simulink model "Lab6_3"  (R2021a)
settings: Solver=VariableStepAuto  StartTime=0.0  StopTime=.07  RelTol=1e-3  EnableMultiTasking=on
libraries: spsIGBTDiodeLib x8, spsDCVoltageSourceLib x2, spsTriangleGeneratorLib x2, spsSeriesRLCBranchLib x1, spsVoltageMeasurementLib x1, spspowerguiLib x1
settings Model: Creator=usee  LastModifiedBy=User
settings SolverCC: AlgebraicLoopSolver=TrustRegion
settings DataIOCC: ReturnWorkspaceOutputs=off
settings OptimizationCC: LifeSpan=inf
settings DebuggingCC: SFUnexpectedBacktrackingDiag=warning  SFNoUnconditionalDefaultTransitionDiag=warning  SFMachineParentedDataDiag=warning  ArithmeticOperatorsInVariantConditions=warning
settings SFSimCC: SimUseLocalCustomCode=off  CustomCodeUndefinedFunction=UseInterfaceOnly
settings RTWCC: RTWUseLocalCustomCode=off
settings CodeAppCC: StateflowObjectComments=on
settings GRTTargetCC: TargetLangStandard=C89/C90 (ANSI)
settings ConfigComp: CovMetricSettings=dw  CovSaveCumulativeToWorkspaceVar=on  CovSaveSingleToWorkspaceVar=on  CovExternalEMLEnable=off
settings SimscapeCC: SimscapeNormalizeSystem=off

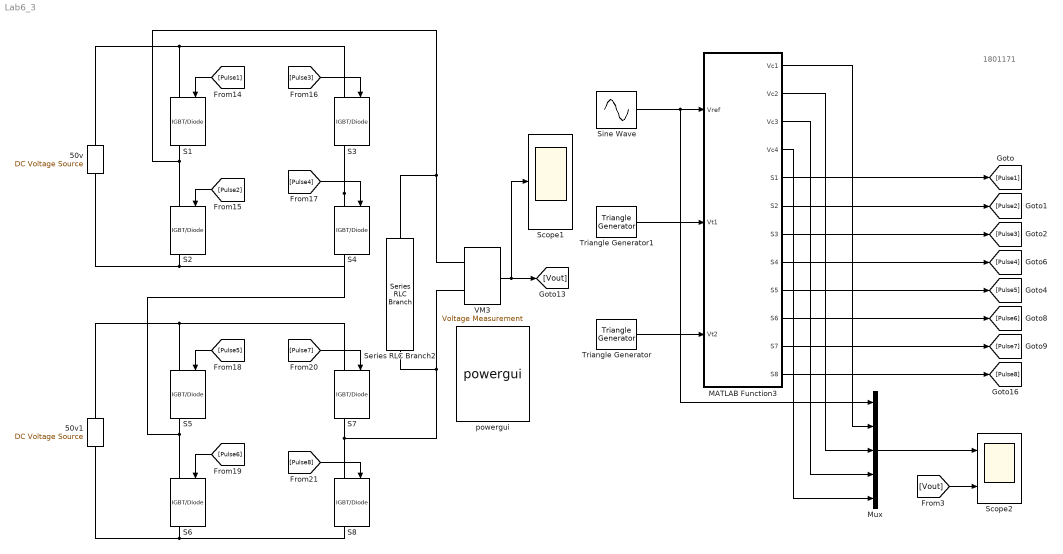
== system Lab6_3 ==
  note: 1801171
  50v : spsDCVoltageSourceLib/DC Voltage Source  Amplitude=50  Measurements=None
  50v1 : spsDCVoltageSourceLib/DC Voltage Source  Amplitude=50  Measurements=None
  MATLAB Function3 : MATLAB Function  TreatAsAtomicUnit=on
  Mux : Mux  Inputs=5
  S{1..8} (8 alike) : spsIGBTDiodeLib/IGBT//Diode  Ron=1e-3  Rs=1e5  Cs=inf  Measurements=on
  Scope1 : Scope
  Scope2 : Scope  NumInputPorts=2
  Series RLC Branch2 : spsSeriesRLCBranchLib/Series RLC Branch  LConnTagsString=__new0  RConnTagsString=__new0  BranchType=RL  Resistance=5  Inductance=10e-3  SetiL0=off  InitialCurrent=0  Capacitance=1e-6  Setx0=off  InitialVoltage=0  Measurements=None
  Sine Wave : Sin  Frequency=2*pi*50  SampleTime=0
  Triangle Generator : spsTriangleGeneratorLib/Triangle Generator  Freq=1000  Phase=0  Ts=0
  Triangle Generator1 : spsTriangleGeneratorLib/Triangle Generator  Freq=1000  Phase=180  Ts=0
  VM3 : spsVoltageMeasurementLib/Voltage Measurement  PhasorSimulation=off  OutputType=Complex  PSBequivalent=0
  powergui : spspowerguiLib/powergui  Priority=1  SimulationMode=Discrete  SampleTime=50e-6  frequency=60  Iterations=50  frequencyindice=0  Pbase=100e6  ErrMax=1e-4  UnitsV=kV  UnitsW=MW  buscounter=0  FunctionMessages=off  echomessages=off  EnableUseOfTLC=off  CurrentSourceSwitches=off  DisableSnubberDevices=off  DisableRonSwitches=off  DisableVfSwitches=off  DisplayEquations=off  AutomaticDiscreteSolvers=off  SolverType=Tustin/Backward Euler (TBE)  Interpol=off  ExternalGateDelay=off  methode=off  Ts=10  x0status=blocks  SPID=off  SwTol=0  HookPort=off  NonlinearTolerance=1e-4  nMaxIteration=100  ContinueOnMaxIteration=off  RestoreLinks=warning  ResistiveCurrentMeasurement=off  Frange=[0:2:500]  Ylog=off  Xlog=on  ShowGrid=off  save=off  variable=ZData  structure=I  ZoomFFT=on  StartTime=0.2  cycles=5  DisplayStyle=2  fundamental=50  FreqAxis=off  MaxFrequency=1000  frequencyindicesteady=1  RmsSteady=1  display=off
  wires:
  MATLAB Function3/5(S1) -> [Pulse1]
  MATLAB Function3/6(S2) -> [Pulse2]
  MATLAB Function3/7(S3) -> [Pulse3]
  MATLAB Function3/8(S4) -> [Pulse4]
  [Vout] -> Scope2/2
  VM3/1 -> [Vout], Scope1/1
  Triangle Generator/1 -> MATLAB Function3/3(Vt2)
  MATLAB Function3/12(S8) -> [Pulse8]
  MATLAB Function3/11(S7) -> [Pulse7]
  MATLAB Function3/10(S6) -> [Pulse6]
  MATLAB Function3/9(S5) -> [Pulse5]
  [Pulse1] -> S1/1
  [Pulse2] -> S2/1
  [Pulse3] -> S3/1
  [Pulse4] -> S4/1
  [Pulse5] -> S5/1
  [Pulse7] -> S7/1
  [Pulse6] -> S6/1
  [Pulse8] -> S8/1
  Sine Wave/1 -> MATLAB Function3/1(Vref), Mux/1
  Mux/1 -> Scope2/1
  Triangle Generator1/1 -> MATLAB Function3/2(Vt1)
  MATLAB Function3/1(Vc1) -> Mux/2
  MATLAB Function3/2(Vc2) -> Mux/3
  MATLAB Function3/3(Vc3) -> Mux/4
  MATLAB Function3/4(Vc4) -> Mux/5
  connections:
  S3/LConn1 -- 50v/RConn1 -- S1/LConn1
  S4/RConn1 -- 50v/LConn1 -- S2/RConn1
  S5/RConn1 -- S3/RConn1 -- S4/LConn1 -- S6/LConn1
  S5/LConn1 -- 50v1/RConn1 -- S7/LConn1
  50v1/LConn1 -- S8/RConn1 -- S6/RConn1
  S8/LConn1 -- VM3/LConn2 -- Series RLC Branch2/RConn1 -- S7/RConn1
  S1/RConn1 -- Series RLC Branch2/LConn1 -- VM3/LConn1 -- S2/LConn1

== matlab function Lab6_3/MATLAB Function3 ==
  data: Vc1 output; Vc2 output; Vc3 output; Vc4 output; Vref input; S1 output; Vt1 input; Vt2 input; S2 output; S3 output; S4 output; S5 output; S6 output; S7 output; S8 output
function [Vc1, Vc2, Vc3, Vc4, S1, S2, S3, S4, S5, S6, S7, S8] = fcn(Vref, Vt1, Vt2)
Vc1 = (Vt1+1)*.25
Vc2 = .5+((Vt1+1)*.25)
Vc3 = (Vt2-1)*.25
Vc4 = -0.5+((Vt2-1)*.25)
if Vref>=0
if Vref>=0 && Vref<=0.5
    if  Vref>=Vc1
        S1=1; S2=0; S3=0; S4=1;
        S5=1; S6=0; S7=1; S8=0;
    else
        S1=1; S2=0; S3=1; S4=0; 
        S5=1; S6=0; S7=1; S8=0;
    end
else Vref>0.5 && Vref<=1
     if  Vref>=Vc2
        S1=1; S2=0; S3=0; S4=1;
        S5=1; S6=0; S7=0; S8=1;
    else
       S1=1; S2=0; S3=0; S4=1;
       S5=1; S6=0; S7=1; S8=0;
     end
end

else
if Vref<0 && Vref>=-0.5
    if  Vref<=Vc3
        S1=0; S2=1; S3=1; S4=0;
        S5=1; S6=0; S7=1; S8=0;
    else
        S1=1; S2=0; S3=1; S4=0; 
        S5=1; S6=0; S7=1; S8=0;
    end
else Vref<-0.5 && Vref>=-1
     if  Vref<=Vc4
        S1=0; S2=1; S3=1; S4=0;
        S5=0; S6=1; S7=1; S8=0;
    else
       S1=0; S2=1; S3=1; S4=0;
       S5=1; S6=0; S7=1; S8=0;
     end
end
end
end
